simulink model "sfcndemo_sfun_errhdl"  (Simulink 7.6)
settings: Solver=FixedStepDiscrete  StartTime=0.0  StopTime=10.0  RelTol=1e-3
Description:
  | Error Handling in Parameters of a C-MEX S-function
settings Model: Creator=The MathWorks Inc.  ExtModeTrigMode=oneshot  ExtModeArmWhenConnect=off  ExtModeAutoUpdateStatusClock=off
settings DataIOCC: LimitDataPoints=off
settings OptimizationCC: BlockReduction=off  BooleanDataType=off  InlineInvariantSignals=on  InitFltsAndDblsToZero=on
settings DebuggingCC: SaveWithParameterizedLinksMsg=none  SignalResolutionControl=TryResolveAllWithWarning  SolverPrmCheckMsg=none  MultiTaskDSMMsg=warning  MultiTaskCondExecSysMsg=none
settings HardwareCC: TargetUnknown=on
settings RTWCC: IncludeERTFirstTime=on
settings CodeAppCC: CustomSymbolStrFcn=$F$N$M
settings GRTTargetCC: TargetFcnLib=ansi_tfl_tmw.mat

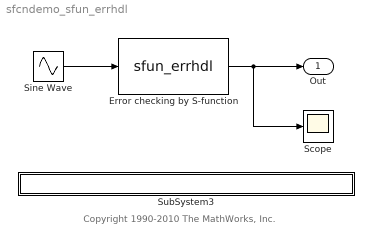
== system sfcndemo_sfun_errhdl ==
  note: Copyright 1990-2010 The MathWorks, Inc.
  Error checking by S-function : S-Function  FunctionName=sfun_errhdl  Parameters=param  EnableBusSupport=off  mask(S-function: sfun_errhdl){param=2.3}
      mask prompts: param "Input parameter:"
      mask help: An example of handling parameter checking in S-function.
      mask Display: disp('Error\nHandling');
  Scope : Scope
      settings: TickLabels=on  TimeRange=10  YMin=-3  YMax=3  DataFormat=Array
  Sine Wave : Sin  SampleTime=0
  SubSystem3 : Subsystem  mask{filename=sfun_errhdl.c}
      mask init:
      | x=sfundemo_maskdisp;
      settings: AttributesFormatString=\n  OpenFcn=sfundemo_openfcn
      mask Display: disp(x);
  Out : Outport  InitialOutput=0
  wires:
  Sine Wave/1 -> Error checking by S-function/1
  Error checking by S-function/1 -> Out/1, Scope/1

== system sfcndemo_sfun_errhdl/SubSystem3 ==
